simulink model "Fuel_filter"  (R2019a)
settings: Solver=FixedStepAuto  StartTime=0.0  StopTime=10.0  FixedStep=1  RelTol=1e-3
settings Model: Creator=Akshay  LastModifiedBy=Akshay

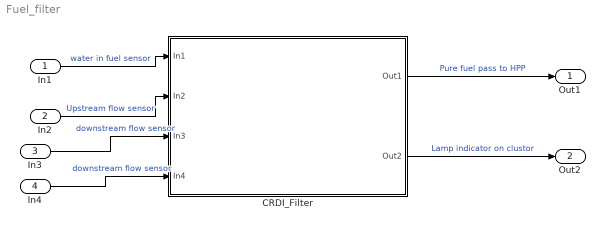
== system Fuel_filter ==
  In1 : Inport
  In2 : Inport  Port=2
  In3 : Inport  Port=3
  In4 : Inport  Port=4
  CRDI_Filter : Subsystem
  Out1 : Outport
  Out2 : Outport  Port=2
  wires:
  CRDI_Filter/1(Out1) -> Out1/1  "Pure fuel pass to HPP"
  CRDI_Filter/2(Out2) -> Out2/1  "Lamp indicator on clustor"
  In1/1 -> CRDI_Filter/1(In1)  "water in fuel sensor"
  In3/1 -> CRDI_Filter/3(In3)  "downstream flow sensor"
  In2/1 -> CRDI_Filter/2(In2)  "Upstream flow sensor"
  In4/1 -> CRDI_Filter/4(In4)  "downstream flow sensor"

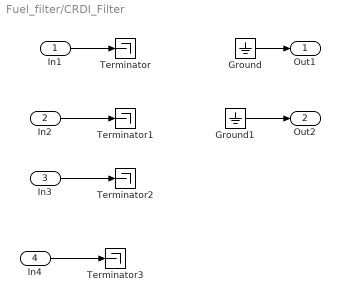
== system Fuel_filter/CRDI_Filter ==
  In1 : Inport
  In2 : Inport  Port=2
  In3 : Inport  Port=3
  In4 : Inport  Port=4
  Ground : Ground
  Ground1 : Ground
  Terminator{,1..3} (4 alike) : Terminator
  Out1 : Outport
  Out2 : Outport  Port=2
  wires:
  In1/1 -> Terminator/1
  In2/1 -> Terminator1/1
  Ground/1 -> Out1/1
  Ground1/1 -> Out2/1
  In3/1 -> Terminator2/1
  In4/1 -> Terminator3/1
